simulink model "T_Junction_middel"  (R2021a)
settings: Solver=VariableStepAuto  StartTime=0.0  StopTime=10.0  RelTol=1e-3
libraries: StreetLanesLibrary x6
settings Model: Creator=timyb  LastModifiedBy=timyb

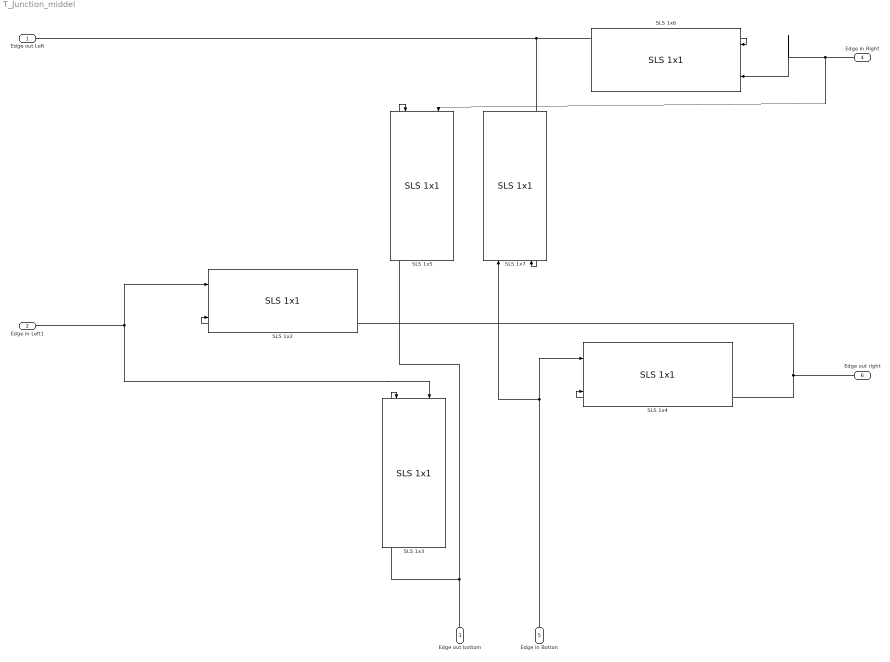
== system T_Junction_middel ==
  Edge out Left : Inport
  Edge in Left1 : Inport  Port=2
  Edge out bottom : Inport  Port=3
  Edge in Right : Inport  Port=4
  Edge in Botton : Inport  Port=5
  Edge out right : Inport  Port=6
  SLS 1x{2..7} (6 alike) : StreetLanesLibrary/SLS 1x1  Kz=0  Tz=0
  wires:
  Edge in Left1/1 -> SLS 1x3/1, SLS 1x2/1
  Edge out Left/1 -> SLS 1x7/2, SLS 1x6/2
  Edge out bottom/1 -> SLS 1x5/2, SLS 1x3/2
  Edge in Right/1 -> SLS 1x5/1, SLS 1x6/1
  Edge in Botton/1 -> SLS 1x7/1, SLS 1x4/1
  Edge out right/1 -> SLS 1x4/2, SLS 1x2/2
